simulink model "Only_dynamic_with_slip"  (R2020a)
settings: Solver=VariableStepAuto  StartTime=0.0  StopTime=10.0  RelTol=1e-3
values from neighbouring files (symbols this model uses):
  b = 0.05    [Dynamics_without_slip_test.m]    (also in Simulate_dynamics_with_slip.m)
  Iwy = 0.025    [Dynamics_without_slip_test.m]    (also in Simulate_dynamics_with_slip.m = 0.0025)
  K = 0.8    [Dynamics_without_slip_test.m]    (also in Simulate_dynamics_with_slip.m = 0.7)
  L = 0.164    [Dynamics_without_slip_test.m]    (also in Simulate_dynamics_with_slip.m)
  mr = mc    (= 2)    [Dynamics_without_slip_test.m]    (also in Simulate_dynamics_with_slip.m)
  P1 = (Ic + 2*Iwy + L^2*mr + 4*b^2*mw + b^2*mr)    (= 0.845792)    [Dynamics_without_slip_test.m]    (also in Formulating_controller.m = (Ic + 2*Iwy + L^2*mr + 4*b^2*mw + b^2*mr); Simulate_dynamics_with_slip.m = 6.77369882864)
  P2 = (- mr*b^2 + mr*L^2 + Ic + 2*Iwy)    (= 0.830792)    [Dynamics_without_slip_test.m]    (also in Formulating_controller.m = -(- mr*b^2 + mr*L^2 + Ic + 2*Iwy); Simulate_dynamics_with_slip.m = 0.867793403695)
  r = 0.0364    [Simulate_dynamics_with_slip.m]
settings Model: Creator=Omkar  LastModifiedBy=Omkar

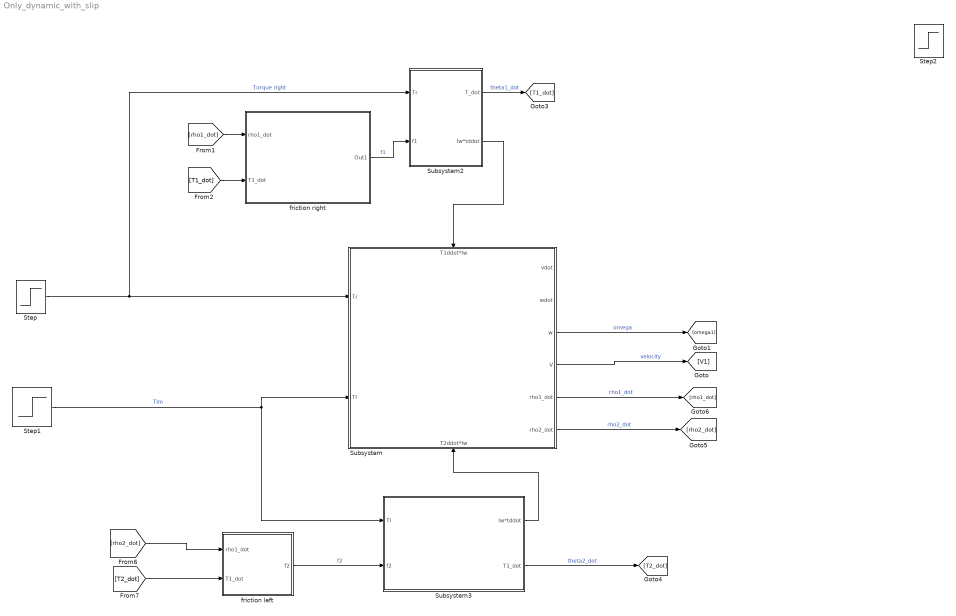
== system Only_dynamic_with_slip ==
  Step : Step  SampleTime=0
  Step1 : Step  After=-1  SampleTime=0
  Step2 : Step  SampleTime=0
  Subsystem : Subsystem
      settings: PortSchema="{\"entries\":[{\"content\":{\"sides\":[{\"content\":{\"connectorIds\":[\"In1\",\"In2\"]},\"type\":\"ConnectorPlacement.EquallySpacedRectSide\",\"uuid\":\"0f741662-0aa0-4f70-a7bc-4d81cf189765\"},{\"content\":{\"connectorIds\":[\"Out1\",\"Out2\",\"Out3\",\"Out4\",\"Out5\",\"Out6\"],\"side\":\"RIGHT\"},\"type\":\"ConnectorPlacement.EquallySpacedRectSide\",\"uuid\":\"61345bba-0f4e-4a45-813f-191783faa34f\"},{\"content\":{\"connectorIds\":[\"In3\"],\"side\":\"TOP\"},\"type\":\"ConnectorPlacement.EquallySpacedRectSide\",\"uuid\":\"0103c91a-592f-4929-b07b-fba43ce48b45\"},{\"content\":{\"connectorIds\":[\"In4\"],\"side\":\"BOTTOM\"},\"type\":\"ConnectorPlacement.EquallySpacedRectSide\",\"uuid\":\"68c4f66e-e2f5-4800-b564-65a852589ef9\"}]},\"type\":\"ConnectorPlacement.EquallySpacedConnector\",\"uuid\":\"b6bd52cb-c94d-4866-979c-ba78b8ff4ad7\"}],\"packageUris\":[\"http://schema.mathworks.com/mf0/Connector/19700101\"],\"version\":\"1.0\"}"
  Subsystem2 : Subsystem
      settings: PortSchema="{\"entries\":[{\"content\":{\"sides\":[{\"content\":{\"connectorIds\":[]},\"type\":\"ConnectorPlacement.EquallySpacedRectSide\",\"uuid\":\"87b04e3d-c928-480c-a1a1-1313223c5e38\"},{\"content\":{\"connectorIds\":[],\"side\":\"RIGHT\"},\"type\":\"ConnectorPlacement.EquallySpacedRectSide\",\"uuid\":\"24b15049-813d-4502-a6fe-723c7c9acef1\"},{\"content\":{\"connectorIds\":[\"In1\",\"In2\"],\"side\":\"TOP\"},\"type\":\"ConnectorPlacement.EquallySpacedRectSide\",\"uuid\":\"f1eb58bb-616f-4565-a8fb-035afd9aaf22\"},{\"content\":{\"connectorIds\":[\"Out1\",\"Out2\"],\"side\":\"BOTTOM\"},\"type\":\"ConnectorPlacement.EquallySpacedRectSide\",\"uuid\":\"8c9ba54b-72de-4f17-9163-80eba6f391e2\"}]},\"type\":\"ConnectorPlacement.EquallySpacedConnector\",\"uuid\":\"ee8d76b6-d516-4cd3-af23-8bf5520b64c4\"}],\"packageUris\":[\"http://schema.mathworks.com/mf0/Connector/19700101\"],\"version\":\"1.0\"}"
  Subsystem3 : Subsystem
      settings: PortSchema="{\"entries\":[{\"content\":{\"sides\":[{\"content\":{\"connectorIds\":[]},\"type\":\"ConnectorPlacement.EquallySpacedRectSide\",\"uuid\":\"87b04e3d-c928-480c-a1a1-1313223c5e38\"},{\"content\":{\"connectorIds\":[],\"side\":\"RIGHT\"},\"type\":\"ConnectorPlacement.EquallySpacedRectSide\",\"uuid\":\"24b15049-813d-4502-a6fe-723c7c9acef1\"},{\"content\":{\"connectorIds\":[\"In1\",\"In2\"],\"side\":\"TOP\"},\"type\":\"ConnectorPlacement.EquallySpacedRectSide\",\"uuid\":\"f1eb58bb-616f-4565-a8fb-035afd9aaf22\"},{\"content\":{\"connectorIds\":[\"Out1\",\"Out2\"],\"side\":\"BOTTOM\"},\"type\":\"ConnectorPlacement.EquallySpacedRectSide\",\"uuid\":\"46d851b4-e0d9-4136-8fd7-44bf774a519f\"}]},\"type\":\"ConnectorPlacement.EquallySpacedConnector\",\"uuid\":\"ee8d76b6-d516-4cd3-af23-8bf5520b64c4\"}],\"packageUris\":[\"http://schema.mathworks.com/mf0/Connector/19700101\"],\"version\":\"1.0\"}"
  friction left : Subsystem
  friction right : Subsystem
  wires:
  Step/1 -> Subsystem2/1(Tr), Subsystem/1(Tr)  "Torque right"
  friction right/1(Out1) -> Subsystem2/2(f1)  "f1"
  friction left/1(f2) -> Subsystem3/2(f2)  "f2"
  [T1_dot] -> friction right/2(T1_dot)
  Subsystem/3(w) -> [omega1]  "omega"
  [T2_dot] -> friction left/2(T1_dot)
  Subsystem/6("rho2_dot ") -> [rho2_dot]  "rho2_dot"
  Subsystem/5(rho1_dot) -> [rho1_dot]  "rho1_dot"
  Subsystem3/1(Iw*tddot) -> Subsystem/4(T2ddot*Iw)
  [rho2_dot] -> friction left/1(rho1_dot)
  Subsystem3/2(T1_dot) -> [T2_dot]  "theta2_dot"
  Subsystem2/2(Iw*tddot) -> Subsystem/3(T1ddot*Iw)
  Step1/1 -> Subsystem/2(Tl), Subsystem3/1(Tl)  "Tlm"
  Subsystem2/1(T_dot) -> [T1_dot]  "theta1_dot"
  [rho1_dot] -> friction right/1(rho1_dot)
  Subsystem/4(V) -> [V1]  "velocity"

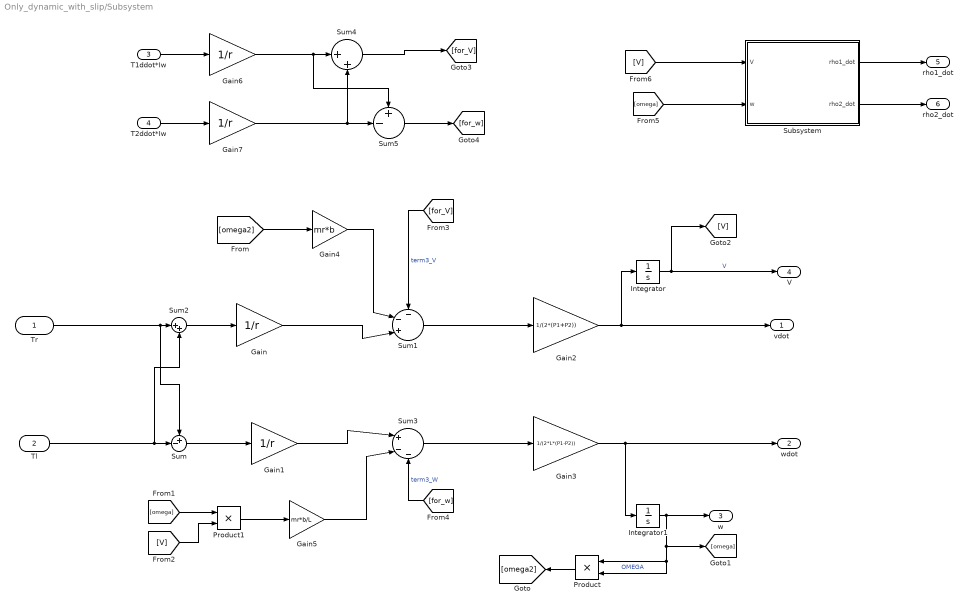
== system Only_dynamic_with_slip/Subsystem ==
  Tr : Inport
  Tl : Inport  Port=2
  T1ddot*Iw : Inport  Port=3
  T2ddot*Iw : Inport  Port=4
  Gain{,1,6..7} (4 alike) : Gain  Gain=1/r
  Gain2 : Gain  Gain=1/(2*(P1+P2))
  Gain3 : Gain  Gain=1/(2*L*(P1-P2))
  Gain4 : Gain  Gain=mr*b
  Gain5 : Gain  Gain=mr*b/L
  Integrator : Integrator
  Integrator1 : Integrator
  Product : Product
  Product1 : Product
  Subsystem : Subsystem
  Sum : Sum  Inputs=+-|
  Sum1 : Sum  Inputs=--+|
  Sum2 : Sum  Inputs=|++
  Sum3 : Sum  Inputs=|+--
  Sum4 : Sum  Inputs=|++
  Sum5 : Sum  Inputs=+-|
  vdot : Outport
  wdot : Outport  Port=2
  w : Outport  Port=3
  V : Outport  Port=4
  rho1_dot : Outport  Port=5
  "rho2_dot " : Outport  Port=6
  wires:
  Tr/1 -> Sum/1, Sum2/1
  Tl/1 -> Sum/2, Sum2/2
  Sum2/1 -> Gain/1
  Sum/1 -> Gain1/1
  Gain3/1 -> Integrator1/1, wdot/1
  Gain2/1 -> Integrator/1, vdot/1
  Integrator/1 -> [V], V/1  "V"
  Integrator1/1 -> [omega], Product/1, Product/2, w/1  "OMEGA"
  Product/1 -> [omega2]
  [omega2] -> Gain4/1
  Gain/1 -> Sum1/3
  Gain4/1 -> Sum1/2
  Gain1/1 -> Sum3/1
  Gain5/1 -> Sum3/2
  Product1/1 -> Gain5/1
  [omega] -> Product1/1
  [V] -> Product1/2
  T1ddot*Iw/1 -> Gain6/1
  T2ddot*Iw/1 -> Gain7/1
  Gain6/1 -> Sum5/1, Sum4/1
  Gain7/1 -> Sum5/2, Sum4/2
  Sum4/1 -> [for_V]
  Sum5/1 -> [for_w]
  [for_V] -> Sum1/1  "term3_V"
  Sum1/1 -> Gain2/1
  [for_w] -> Sum3/3  "term3_W"
  Sum3/1 -> Gain3/1
  [V] -> Subsystem/1(V)
  [omega] -> Subsystem/2(w)
  Subsystem/1(rho1_dot) -> rho1_dot/1
  Subsystem/2("rho2_dot ") -> "rho2_dot "/1

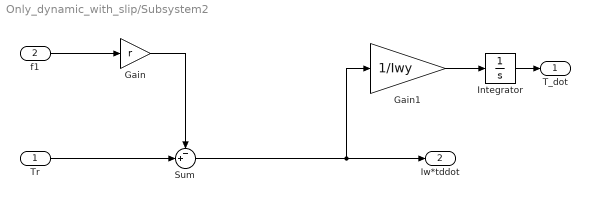
== system Only_dynamic_with_slip/Subsystem2 ==
  Tr : Inport
  f1 : Inport  Port=2
  Gain : Gain  Gain=r
  Gain1 : Gain  Gain=1/Iwy
  Integrator : Integrator
  Sum : Sum  Inputs=-+|
  T_dot : Outport
  Iw*tddot : Outport  Port=2
  wires:
  Tr/1 -> Sum/2
  Gain/1 -> Sum/1
  f1/1 -> Gain/1
  Integrator/1 -> T_dot/1
  Sum/1 -> Iw*tddot/1, Gain1/1
  Gain1/1 -> Integrator/1

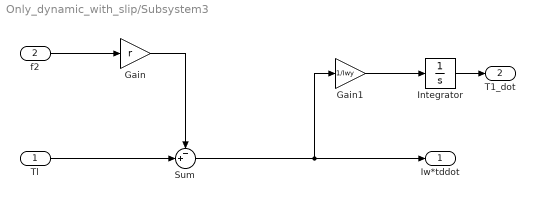
== system Only_dynamic_with_slip/Subsystem3 ==
  Tl : Inport
  f2 : Inport  Port=2
  Gain : Gain  Gain=r
  Gain1 : Gain  Gain=1/Iwy
  Integrator : Integrator
  Sum : Sum  Inputs=-+|
  Iw*tddot : Outport
  T1_dot : Outport  Port=2
  wires:
  Tl/1 -> Sum/2
  Gain/1 -> Sum/1
  f2/1 -> Gain/1
  Sum/1 -> Gain1/1, Iw*tddot/1
  Integrator/1 -> T1_dot/1
  Gain1/1 -> Integrator/1

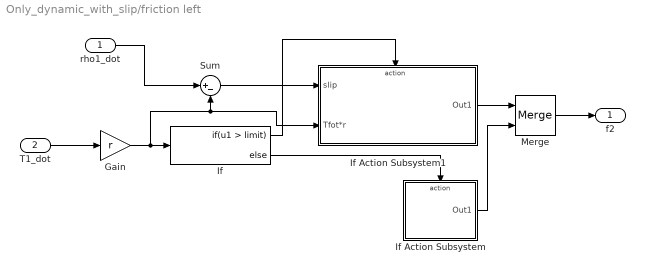
== system Only_dynamic_with_slip/friction left ==
  rho1_dot : Inport
  T1_dot : Inport  Port=2
  Gain : Gain  Gain=r
  If : If  IfExpression=u1 > limit
  If Action Subsystem : Subsystem  TreatAsAtomicUnit=on
  If Action Subsystem1 : Subsystem  TreatAsAtomicUnit=on
  Merge : Merge
  Sum : Sum  Inputs=|+-
  f2 : Outport
  wires:
  If/2 -> If Action Subsystem/Action
  If/1 -> If Action Subsystem1/Action
  Sum/1 -> If Action Subsystem1/1(slip)
  If Action Subsystem1/1(Out1) -> Merge/1
  If Action Subsystem/1(Out1) -> Merge/2
  T1_dot/1 -> Gain/1
  Gain/1 -> Sum/2, If Action Subsystem1/2(Tfot*r), If/1
  Merge/1 -> f2/1
  rho1_dot/1 -> Sum/1

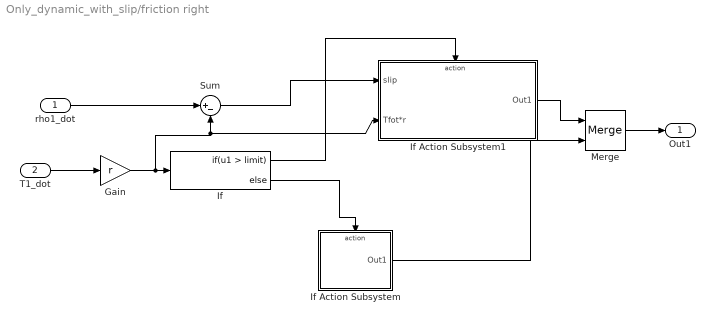
== system Only_dynamic_with_slip/friction right ==
  rho1_dot : Inport
  T1_dot : Inport  Port=2
  Gain : Gain  Gain=r
  If : If  IfExpression=u1 > limit
  If Action Subsystem : Subsystem  TreatAsAtomicUnit=on
  If Action Subsystem1 : Subsystem  TreatAsAtomicUnit=on
  Merge : Merge
  Sum : Sum  Inputs=|+-
  Out1 : Outport
  wires:
  Merge/1 -> Out1/1
  T1_dot/1 -> Gain/1
  If Action Subsystem/1(Out1) -> Merge/2
  If Action Subsystem1/1(Out1) -> Merge/1
  rho1_dot/1 -> Sum/1
  Sum/1 -> If Action Subsystem1/1(slip)
  If/1 -> If Action Subsystem1/Action
  If/2 -> If Action Subsystem/Action
  Gain/1 -> If Action Subsystem1/2(Tfot*r), Sum/2, If/1

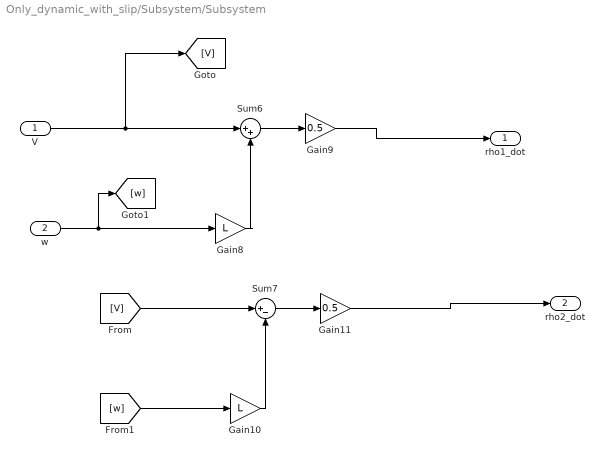
== system Only_dynamic_with_slip/Subsystem/Subsystem ==
  V : Inport
  w : Inport  Port=2
  Gain10 : Gain  Gain=L
  Gain11 : Gain  Gain=0.5
  Gain8 : Gain  Gain=L
  Gain9 : Gain  Gain=0.5
  Sum6 : Sum  Inputs=|++
  Sum7 : Sum  Inputs=|+-
  rho1_dot : Outport
  "rho2_dot " : Outport  Port=2
  wires:
  Gain11/1 -> "rho2_dot "/1
  Gain9/1 -> rho1_dot/1
  V/1 -> [V], Sum6/1
  Gain8/1 -> Sum6/2
  Sum6/1 -> Gain9/1
  Sum7/1 -> Gain11/1
  Gain10/1 -> Sum7/2
  [w] -> Gain10/1
  w/1 -> [w], Gain8/1
  [V] -> Sum7/1

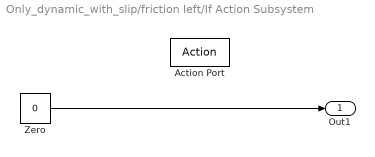
== system Only_dynamic_with_slip/friction left/If Action Subsystem ==
  Action Port : ActionPort  ActionPortLabel=else
  Zero : Constant  Value=0  OutDataTypeStr=Inherit: Inherit via back propagation
  Out1 : Outport
  wires:
  Zero/1 -> Out1/1

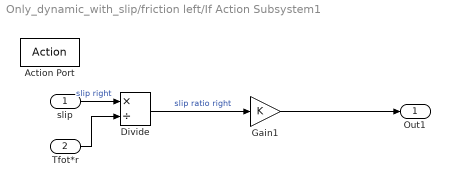
== system Only_dynamic_with_slip/friction left/If Action Subsystem1 ==
  slip : Inport
  Tfot*r : Inport  Port=2
  Action Port : ActionPort  ActionPortLabel=if(u1 > limit)
  Divide : Product  Inputs=*/  RndMeth=Zero  SaturateOnIntegerOverflow=on
  Gain1 : Gain  Gain=K
  Out1 : Outport
  wires:
  Gain1/1 -> Out1/1
  Tfot*r/1 -> Divide/2
  Divide/1 -> Gain1/1  "slip ratio right"
  slip/1 -> Divide/1  "slip right"

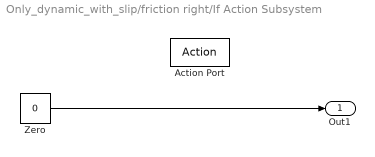
== system Only_dynamic_with_slip/friction right/If Action Subsystem ==
  Action Port : ActionPort  ActionPortLabel=else
  Zero : Constant  Value=0  OutDataTypeStr=Inherit: Inherit via back propagation
  Out1 : Outport
  wires:
  Zero/1 -> Out1/1

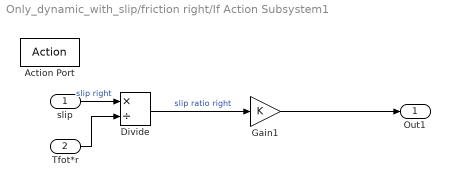
== system Only_dynamic_with_slip/friction right/If Action Subsystem1 ==
  slip : Inport
  Tfot*r : Inport  Port=2
  Action Port : ActionPort  ActionPortLabel=if(u1 > limit)
  Divide : Product  Inputs=*/  RndMeth=Zero  SaturateOnIntegerOverflow=on
  Gain1 : Gain  Gain=K
  Out1 : Outport
  wires:
  Gain1/1 -> Out1/1
  Tfot*r/1 -> Divide/2
  Divide/1 -> Gain1/1  "slip ratio right"
  slip/1 -> Divide/1  "slip right"
